simulink model "untitled2"  (Simulink 8.6)
settings: Solver=ode23tb  StartTime=0.0  StopTime=0.06  MaxStep=1e-5  RelTol=1e-3
libraries: powerlib x6, powerlib_extras x3, simulink x1
settings Model: Creator=HZ  LastModifiedBy=Administrator
settings OptimizationCC: InitFltsAndDblsToZero=on
settings DebuggingCC: SaveWithParameterizedLinksMsg=none  SignalResolutionControl=TryResolveAllWithWarning  MultiTaskDSMMsg=warning  MultiTaskCondExecSysMsg=none  FcnCallInpInsideContextMsg=UseLocalSettings  StrictBusMsg=WarnOnBusTreatedAsVector
settings GRTTargetCC: TargetFcnLib=ansi_tfl_tmw.mat  GeneratePreprocessorConditionals=Use local settings

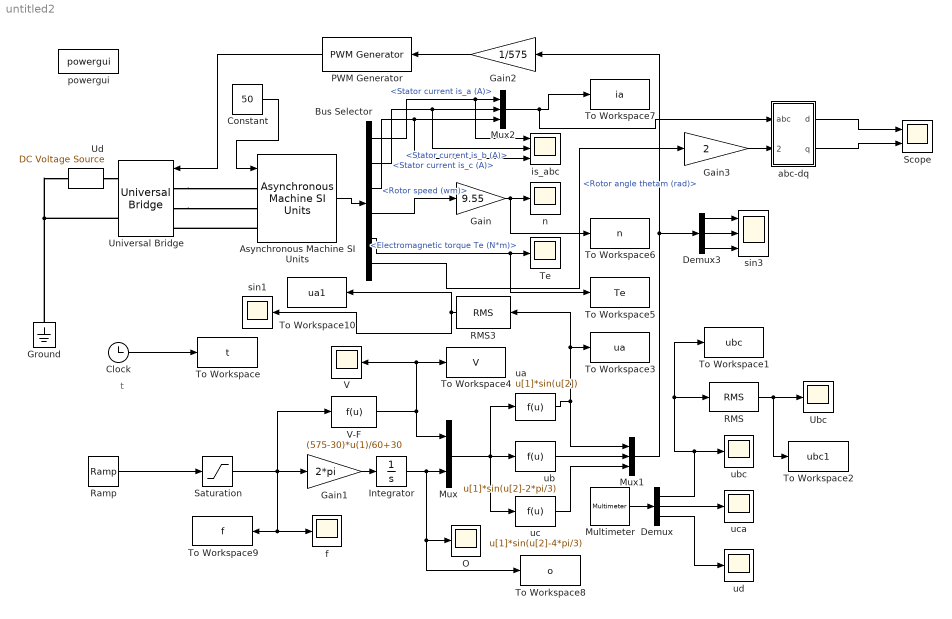
== system untitled2 ==
  note: t
  Asynchronous Machine SI Units : powerlib/Machines/Asynchronous Machine SI Units  RotorType=Squirrel-cage  PresetModel="08:  5 HP   575 V 60Hz 1750 RPM"  MechanicalLoad=Torque Tm  ShowDetailedParameters=on  ReferenceFrame=Rotor  Units=SI  MeasurementBus=off  NominalParameters=[3730 575 60]  Stator=[2.053 0.008101]  Rotor=[1.904 0.008101]  Cage1=[0.4155 0.002066]  Cage2=[0.4168 0.0003495]  Lm=0.3144  Mechanical=[0.02 0.002494 2]  PolePairs=2  InitialConditions="[ 1,0   0,0,0   0,0,0 ]"  SimulateSaturation=off  Saturation=[9.9249,19.6672,38.0377,51.3988,69.2824,105.1337,152.5532,214.2421,303.1917;230, 322, 414, 460, 506, 552, 598, 644, 690]  LoadFlowParameters=0  TsPowergui=0  TsBlock=-1  IterativeModel=Forward Euler  Pmec=1.492e+006
  Bus Selector : BusSelector  OutputSignals=Stator measurements.Stator current is_a (A),Stator measurements.Stator current is_b (A),Stator measurements.Stator current is_c (A),Mechanical.Rotor speed (wm),Mechanical.Electromagnetic torque Te (N*m),Mechanical.Rotor angle thetam (rad)
  Clock : Clock
  Constant : Constant  Value=50
  Demux : Demux  Outputs=3
  Demux3 : Demux  Outputs=3
  Gain : Gain  Gain=9.55
  Gain1 : Gain  Gain=2*pi
  Gain2 : Gain  Gain=1/575
  Gain3 : Gain  Gain=2
  Ground : powerlib/Elements/Ground  LConnTagsString=a
  Integrator : Integrator
  Multimeter : powerlib/Measurements/Multimeter  PhasorSimulation=off  OutputType=Complex  sel=[8 9 11]  L=17  Gain=[1 1 1]  yselected={'Ubc: Universal Bridge','Uca: Universal Bridge','Usrc: Ud'};  PSBOutputType=1  PSBequivalent=0  AxesSetting=[0,0.1,-100,100]  Display=0  SavedBlockNames=-11
  Mux : Mux  Inputs=2
  Mux1 : Mux  Inputs=3
  Mux2 : Mux  Inputs=3
  O : Scope
  PWM Generator : powerlib_extras/Control  Blocks/PWM Generator  GeneratorMode="3-arm  bridge (6 pulses)"  Fc=1800  Internal=off  mIndex=0.4  Freq=60  Phase=0
  RMS : powerlib_extras/Measurements/RMS  f1=60
  RMS3 : powerlib_extras/Measurements/RMS  f1=60
  Ramp : simulink/Sources/Ramp  slope=10  start=0  X0=0
  Saturation : Saturate  UpperLimit=60
  Scope : Scope  NumInputPorts=2
  Te : Scope
  To Workspace : ToWorkspace  VariableName=t  SampleTime=-1
  To Workspace1 : ToWorkspace  VariableName=ubc  SampleTime=-1
  To Workspace10 : ToWorkspace  VariableName=ua1  SampleTime=-1
  To Workspace2 : ToWorkspace  VariableName=ubc1  SampleTime=-1
  To Workspace3 : ToWorkspace  VariableName=ua  SampleTime=-1
  To Workspace4 : ToWorkspace  VariableName=V  SampleTime=-1
  To Workspace5 : ToWorkspace  VariableName=Te  SampleTime=-1
  To Workspace6 : ToWorkspace  VariableName=n  SampleTime=-1
  To Workspace7 : ToWorkspace  VariableName=ia  SampleTime=-1
  To Workspace8 : ToWorkspace  VariableName=o  SampleTime=-1
  To Workspace9 : ToWorkspace  VariableName=f  SampleTime=-1
  Ubc : Scope
  Ud : powerlib/Electrical Sources/DC Voltage Source  Amplitude=720  Measurements=Voltage
  Universal Bridge : powerlib/Power Electronics/Universal Bridge  Arms=3  SnubberResistance=1e5  SnubberCapacitance=inf  Device=IGBT / Diodes  Ron=1e-3  Lon=0  ForwardVoltages="[  0  0  ]"  ForwardVoltage=0  GTOparameters=[ 10e-6 , 20e-6 ]  IGBTparameters=[ 1e-6 , 2e-6 ]  Measurements=All voltages and currents  Measurements_2=None  converterType=Rectifier
  V : Scope
  V-F : Fcn  Expr=(575-30)*u(1)/60+30
  abc-dq : Subsystem
  f : Scope
  is_abc : Scope  NumInputPorts=3
  n : Scope
  powergui : powerlib/powergui  SimulationMode=Continuous  SolverType=Tustin/Backward Euler (TBE)  SampleTime=1e-4  frequency=60  SPID=off  DisableSnubberDevices=off  DisableRonSwitches=off  DisableVfSwitches=off  SwTol=0  DisplayEquations=off  Interpol=off  ExternalGateDelay=off  methode=off  Ts=0  FunctionMessages=off  echomessages=off  HookPort=off  EnableUseOfTLC=off  x0status=blocks  frequencyindice=60  Pbase=100e6  ErrMax=1e-4  Iterations=50  UnitsV=kV  UnitsW=MW  buscounter=0  RestoreLinks=warning  ResistiveCurrentMeasurement=off  Frange=[0:2:500]  Ylog=off  Xlog=on  ShowGrid=off  save=off  variable=ZData  structure=0  ZoomFFT=on  StartTime=0.0  cycles=1  DisplayStyle=1  fundamental=60  FreqAxis=off  MaxFrequency=1000  frequencyindicesteady=1  RmsSteady=1  display=off
  sin1 : Scope
  sin3 : Scope  NumInputPorts=3
  ua : Fcn  Expr=u[1]*sin(u[2])
  ub : Fcn  Expr=u[1]*sin(u[2]-2*pi/3)
  ubc : Scope
  uc : Fcn  Expr=u[1]*sin(u[2]-4*pi/3)
  uca : Scope
  ud : Scope
  wires:
  PWM Generator/1 -> Universal Bridge/1
  Multimeter/1 -> Demux/1
  Demux/2 -> uca/1
  Demux/3 -> ud/1
  Demux/1 -> ubc/1, RMS/1, To Workspace1/1
  RMS/1 -> Ubc/1, To Workspace2/1
  Bus Selector/4 -> Gain/1  "<Rotor speed (wm)>"
  Gain/1 -> n/1, To Workspace6/1
  Bus Selector/5 -> To Workspace5/1, Te/1  "<Electromagnetic torque Te (N*m)>"
  ua/1 -> Mux1/1, To Workspace3/1, RMS3/1
  ub/1 -> Mux1/2
  uc/1 -> Mux1/3
  Gain2/1 -> PWM Generator/1
  Mux1/1 -> Gain2/1, Demux3/1
  Demux3/1 -> sin3/1
  Demux3/2 -> sin3/2
  Demux3/3 -> sin3/3
  Clock/1 -> To Workspace/1
  Ramp/1 -> Saturation/1
  V-F/1 -> Mux/1, V/1, To Workspace4/1
  Gain1/1 -> Integrator/1
  Integrator/1 -> Mux/2, O/1, To Workspace8/1
  RMS3/1 -> sin1/1, To Workspace10/1
  Mux/1 -> ub/1, ua/1, uc/1
  Saturation/1 -> Gain1/1, f/1, To Workspace9/1, V-F/1
  Asynchronous Machine SI Units/1 -> Bus Selector/1
  Bus Selector/1 -> Mux2/1, is_abc/1  "<Stator current is_a (A)>"
  Bus Selector/2 -> Mux2/2, is_abc/2  "<Stator current is_b (A)>"
  Bus Selector/3 -> Mux2/3, is_abc/3  "<Stator current is_c (A)>"
  Mux2/1 -> abc-dq/1(abc), To Workspace7/1
  Constant/1 -> Asynchronous Machine SI Units/1
  Gain3/1 -> abc-dq/2(theta)
  Bus Selector/6 -> Gain3/1  "<Rotor angle thetam (rad)>"
  abc-dq/1(d) -> Scope/1
  abc-dq/2(q) -> Scope/2
  connections:
  Universal Bridge/LConn1 -- Asynchronous Machine SI Units/LConn1
  Universal Bridge/LConn2 -- Asynchronous Machine SI Units/LConn2
  Asynchronous Machine SI Units/LConn3 -- Universal Bridge/LConn3
  Ud/RConn1 -- Universal Bridge/RConn1
  Ground/LConn1 -- Ud/LConn1 -- Universal Bridge/RConn2

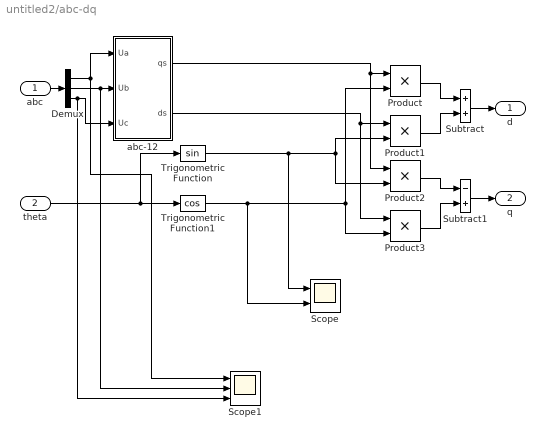
== system untitled2/abc-dq ==
  abc : Inport
  theta : Inport  Port=2
  Demux : Demux  Outputs=3
  Product{,1..3} (4 alike) : Product  RndMeth=Zero
  Scope : Scope  NumInputPorts=2
  Scope1 : Scope  NumInputPorts=3
  Subtract : Sum
  Subtract1 : Sum  Inputs=-+
  Trigonometric Function : Trigonometry
  Trigonometric Function1 : Trigonometry  Operator=cos
  abc-12 : Subsystem
  d : Outport
  q : Outport  Port=2
  wires:
  Demux/3 -> Scope1/3, abc-12/3(Uc)
  Demux/2 -> Scope1/2, abc-12/2(Ub)
  Demux/1 -> abc-12/1(Ua), Scope1/1
  abc/1 -> Demux/1
  abc-12/2(ds) -> Product3/1, Product1/1
  abc-12/1(qs) -> Product2/1, Product/1
  Subtract1/1 -> q/1
  Subtract/1 -> d/1
  Product3/1 -> Subtract1/2
  Product2/1 -> Subtract1/1
  Product1/1 -> Subtract/2
  Product/1 -> Subtract/1
  theta/1 -> Trigonometric Function1/1, Trigonometric Function/1
  Trigonometric Function1/1 -> Scope/2, Product3/2, Product/2
  Trigonometric Function/1 -> Scope/1, Product2/2, Product1/2

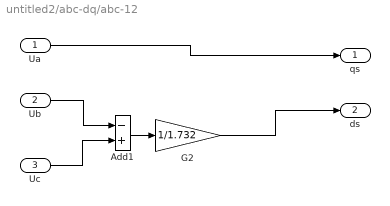
== system untitled2/abc-dq/abc-12 ==
  Ua : Inport
  Ub : Inport  Port=2
  Uc : Inport  Port=3
  Add1 : Sum  Inputs=-+
  G2 : Gain  Gain=1/1.732
  qs : Outport
  ds : Outport  Port=2
  wires:
  Ua/1 -> qs/1
  Ub/1 -> Add1/1
  Uc/1 -> Add1/2
  Add1/1 -> G2/1
  G2/1 -> ds/1
